simulink model "simulink_motor"  (R2018b)
settings: Solver=VariableStepAuto  StartTime=0.0  StopTime=100  RelTol=1e-6
settings Model: Creator=aland  LastModifiedBy=aland

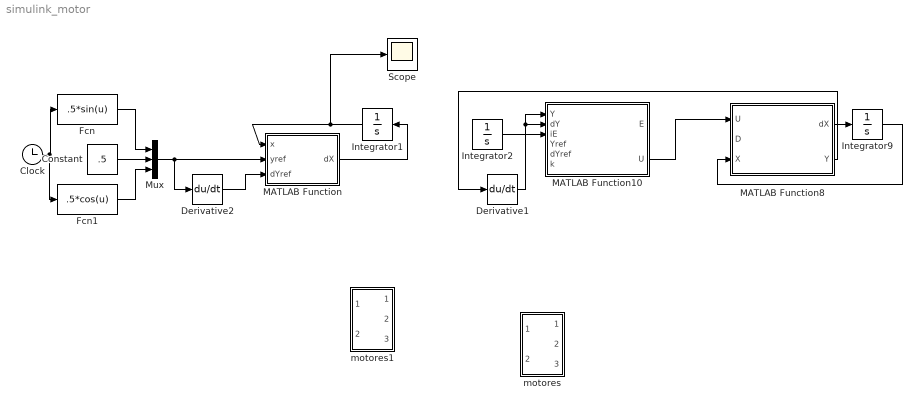
== system simulink_motor ==
  Clock : Clock
      settings: Decimation=1000
  Constant : Constant  Value=.5
  Derivative1 : Derivative
  Derivative2 : Derivative
  Fcn : Fcn  Expr=.5*sin(u)
  Fcn1 : Fcn  Expr=.5*cos(u)
  Integrator1 : Integrator  InitialCondition=[0 0 0 0 0 0 0 .148 0 1.2385]  UpperSaturationLimit=4  LowerSaturationLimit=-4
  Integrator2 : Integrator  InitialCondition=[0 0]
  Integrator9 : Integrator  InitialCondition=[0 0]
  MATLAB Function : MATLAB Function  TreatAsAtomicUnit=on
  MATLAB Function10 : MATLAB Function  TreatAsAtomicUnit=on
  MATLAB Function8 : MATLAB Function  TreatAsAtomicUnit=on
  Mux : Mux  Inputs=3
  Scope : Scope
  motores : Subsystem  InitFcn=robot_init
  motores1 : Subsystem  InitFcn=robot_init
  wires:
  Fcn/1 -> Mux/1
  Constant/1 -> Mux/2
  Fcn1/1 -> Mux/3
  Mux/1 -> Derivative2/1, MATLAB Function/2(yref)
  Derivative2/1 -> MATLAB Function/3(dYref)
  MATLAB Function/1(dX) -> Integrator1/1
  Integrator1/1 -> Scope/1, MATLAB Function/1(x)
  Clock/1 -> Fcn1/1, Fcn/1
  MATLAB Function8/1(dX) -> Integrator9/1
  MATLAB Function10/2(U) -> MATLAB Function8/1(U)
  Integrator9/1 -> MATLAB Function8/3(X)
  MATLAB Function8/2(Y) -> Derivative1/1
  Derivative1/1 -> MATLAB Function10/1(Y), MATLAB Function10/2(dY)
  Integrator2/1 -> MATLAB Function10/3(iE)

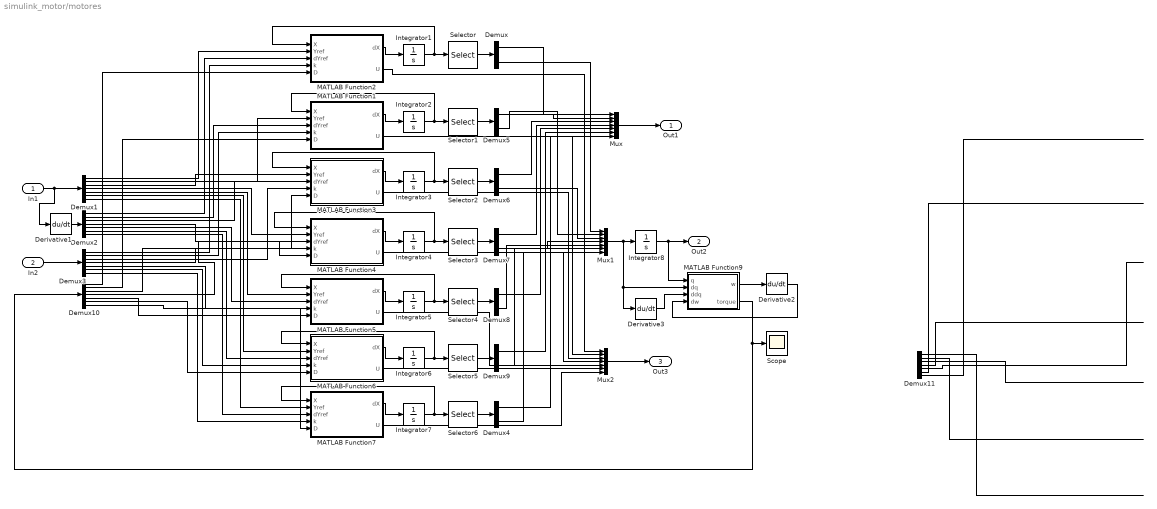
== system simulink_motor/motores ==
  In1 : Inport
  In2 : Inport  Port=2
  Demux{,4..9} (7 alike) : Demux  Outputs=2
  Demux{1..2,10..11} (4 alike) : Demux  Outputs=7
  Demux3 : Demux  Outputs=[3 3 3 3 3 3 3]
  Derivative1 : Derivative
  Derivative2 : Derivative
  Derivative3 : Derivative
  Integrator{1..7} (7 alike) : Integrator  InitialCondition=[0 0 0]
  Integrator8 : Integrator  InitialCondition=[0 0 0 0 0 0 0]  UpperSaturationLimit=4  LowerSaturationLimit=-4
  MATLAB Function1 : MATLAB Function  TreatAsAtomicUnit=on
  MATLAB Function2 : MATLAB Function  TreatAsAtomicUnit=on
  MATLAB Function3 : MATLAB Function  TreatAsAtomicUnit=on
  MATLAB Function4 : MATLAB Function  TreatAsAtomicUnit=on
  MATLAB Function5 : MATLAB Function  TreatAsAtomicUnit=on
  MATLAB Function6 : MATLAB Function  TreatAsAtomicUnit=on
  MATLAB Function7 : MATLAB Function  TreatAsAtomicUnit=on
  MATLAB Function9 : MATLAB Function  TreatAsAtomicUnit=on
      mask init:
      | m = 0;
  Mux : Mux  Inputs=7
  Mux1 : Mux  Inputs=7
  Mux2 : Mux  Inputs=7
  Scope : Scope
  Selector{,1..6} (7 alike) : Selector  InputPortWidth=3  IndexOptions=Index vector (dialog)  Indices=[2:3]  OutputSizes=1
  Out1 : Outport
  Out2 : Outport  Port=2
  Out3 : Outport  Port=3
  wires:
  In2/1 -> Demux3/1
  Demux4/2 -> Mux1/7
  Demux3/6 -> MATLAB Function6/4(k)
  Demux3/2 -> MATLAB Function1/4(k)
  Demux3/4 -> MATLAB Function4/4(k)
  Integrator4/1 -> Selector3/1, MATLAB Function4/1(X)
  Demux5/2 -> Mux1/2
  MATLAB Function3/1(dX) -> Integrator3/1
  MATLAB Function6/1(dX) -> Integrator6/1
  Demux5/1 -> Mux/2
  Integrator2/1 -> Selector1/1, MATLAB Function1/1(X)
  Integrator1/1 -> MATLAB Function2/1(X), Selector/1
  Demux2/7 -> MATLAB Function7/3(dYref)
  MATLAB Function4/1(dX) -> Integrator4/1
  Demux2/1 -> MATLAB Function2/3(dYref)
  Demux3/5 -> MATLAB Function5/4(k)
  Demux1/5 -> MATLAB Function5/2(Yref)
  Integrator6/1 -> Selector5/1, MATLAB Function6/1(X)
  Demux2/3 -> MATLAB Function3/3(dYref)
  Integrator3/1 -> Selector2/1, MATLAB Function3/1(X)
  Demux2/5 -> MATLAB Function5/3(dYref)
  Demux1/4 -> MATLAB Function4/2(Yref)
  MATLAB Function1/1(dX) -> Integrator2/1
  Demux1/6 -> MATLAB Function6/2(Yref)
  Demux7/1 -> Mux/4
  MATLAB Function5/1(dX) -> Integrator5/1
  Integrator5/1 -> Selector4/1, MATLAB Function5/1(X)
  Demux6/1 -> Mux/3
  MATLAB Function7/1(dX) -> Integrator7/1
  Demux1/7 -> MATLAB Function7/2(Yref)
  Demux3/7 -> MATLAB Function7/4(k)
  Demux9/2 -> Mux1/6
  Integrator7/1 -> Selector6/1, MATLAB Function7/1(X)
  Demux1/1 -> MATLAB Function2/2(Yref)
  Demux8/2 -> Mux1/5
  Demux6/2 -> Mux1/3
  Demux3/3 -> MATLAB Function3/4(k)
  Demux7/2 -> Mux1/4
  Demux2/6 -> MATLAB Function6/3(dYref)
  Demux/2 -> Mux1/1
  Demux9/1 -> Mux/6
  Demux8/1 -> Mux/5
  Demux1/2 -> MATLAB Function1/2(Yref)
  Demux/1 -> Mux/1
  Demux1/3 -> MATLAB Function3/2(Yref)
  MATLAB Function2/1(dX) -> Integrator1/1
  Demux3/1 -> MATLAB Function2/4(k)
  Demux2/4 -> MATLAB Function4/3(dYref)
  Demux4/1 -> Mux/7
  Demux2/2 -> MATLAB Function1/3(dYref)
  Mux/1 -> Out1/1
  In1/1 -> Derivative1/1, Demux1/1
  Selector/1 -> Demux/1
  Selector1/1 -> Demux5/1
  Selector2/1 -> Demux6/1
  Selector3/1 -> Demux7/1
  Selector4/1 -> Demux8/1
  Selector5/1 -> Demux9/1
  Selector6/1 -> Demux4/1
  Derivative1/1 -> Demux2/1
  Mux2/1 -> Out3/1
  MATLAB Function2/2(U) -> Mux2/1
  MATLAB Function1/2(U) -> Mux2/2
  MATLAB Function4/2(U) -> Mux2/4
  MATLAB Function3/2(U) -> Mux2/3
  MATLAB Function6/2(U) -> Mux2/6
  MATLAB Function5/2(U) -> Mux2/5
  MATLAB Function7/2(U) -> Mux2/7
  Mux1/1 -> MATLAB Function9/2(dq), Derivative3/1, Integrator8/1
  Integrator8/1 -> MATLAB Function9/1(q), Out2/1
  MATLAB Function9/1(w) -> Derivative2/1
  Derivative2/1 -> MATLAB Function9/4(dw)
  Derivative3/1 -> MATLAB Function9/3(ddq)
  Demux11/1 -> ?
  Demux11/2 -> ?
  Demux11/3 -> ?
  Demux11/4 -> ?
  Demux11/5 -> ?
  Demux11/7 -> ?
  Demux11/6 -> ?
  Demux10/4 -> MATLAB Function4/5(D)
  Demux10/7 -> MATLAB Function7/5(D)
  Demux10/1 -> MATLAB Function2/5(D)
  Demux10/5 -> MATLAB Function5/5(D)
  Demux10/2 -> MATLAB Function1/5(D)
  Demux10/6 -> MATLAB Function6/5(D)
  MATLAB Function9/2(torque) -> Scope/1, Demux10/1
  Demux10/3 -> MATLAB Function3/5(D)

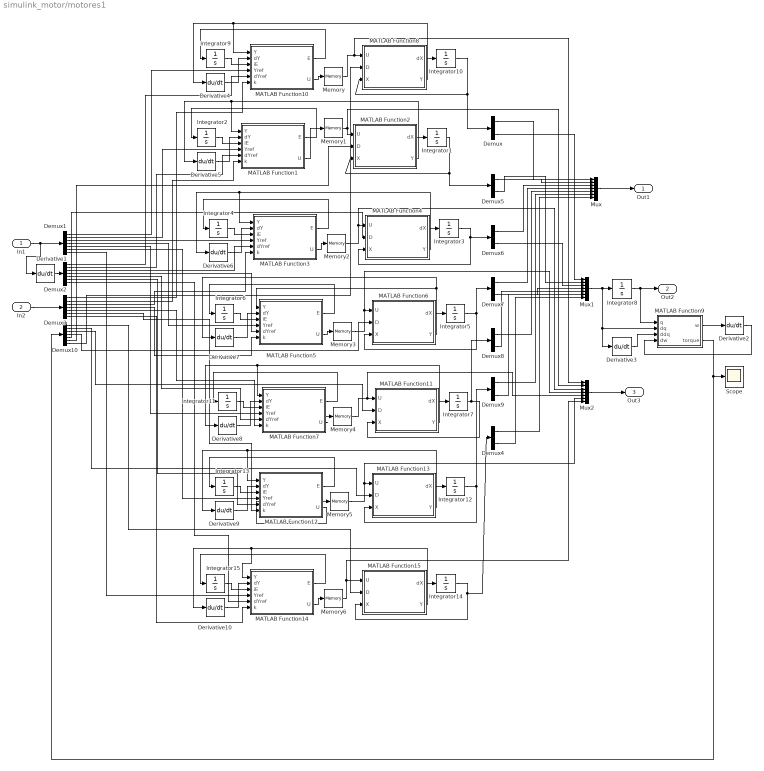
== system simulink_motor/motores1 ==
  In1 : Inport
  In2 : Inport  Port=2
  Demux{,4..9} (7 alike) : Demux  Outputs=2
  Demux1 : Demux  Outputs=7
  Demux10 : Demux  Outputs=7
  Demux2 : Demux  Outputs=7
  Demux3 : Demux  Outputs=[3 3 3 3 3 3 3]
  Derivative{1..10} (10 alike) : Derivative
  Integrator{1,3,5,7,10,12,14} (7 alike) : Integrator  InitialCondition=[0 0]
  Integrator{2,4,6,9,11,13,15} (7 alike) : Integrator
  Integrator8 : Integrator  InitialCondition=[0 0 0 0 0 0 0]  UpperSaturationLimit=4  LowerSaturationLimit=-4
  MATLAB Function1 : MATLAB Function  TreatAsAtomicUnit=on
  MATLAB Function10 : MATLAB Function  TreatAsAtomicUnit=on
  MATLAB Function11 : MATLAB Function  TreatAsAtomicUnit=on
  MATLAB Function12 : MATLAB Function  TreatAsAtomicUnit=on
  MATLAB Function13 : MATLAB Function  TreatAsAtomicUnit=on
  MATLAB Function14 : MATLAB Function  TreatAsAtomicUnit=on
  MATLAB Function15 : MATLAB Function  TreatAsAtomicUnit=on
  MATLAB Function2 : MATLAB Function  TreatAsAtomicUnit=on
  MATLAB Function3 : MATLAB Function  TreatAsAtomicUnit=on
  MATLAB Function4 : MATLAB Function  TreatAsAtomicUnit=on
  MATLAB Function5 : MATLAB Function  TreatAsAtomicUnit=on
  MATLAB Function6 : MATLAB Function  TreatAsAtomicUnit=on
  MATLAB Function7 : MATLAB Function  TreatAsAtomicUnit=on
  MATLAB Function8 : MATLAB Function  TreatAsAtomicUnit=on
  MATLAB Function9 : MATLAB Function  TreatAsAtomicUnit=on
      mask init:
      | m = 0;
  Memory{,1..6} (7 alike) : Memory
  Mux : Mux  Inputs=7
  Mux1 : Mux  Inputs=7
  Mux2 : Mux  Inputs=7
  Scope : Scope
  Out1 : Outport
  Out2 : Outport  Port=2
  Out3 : Outport  Port=3
  wires:
  In2/1 -> Demux3/1
  Demux4/2 -> Mux1/7
  Demux5/2 -> Mux1/2
  Demux5/1 -> Mux/2
  Demux7/1 -> Mux/4
  Demux6/1 -> Mux/3
  Demux9/2 -> Mux1/6
  Demux8/2 -> Mux1/5
  Demux6/2 -> Mux1/3
  Demux7/2 -> Mux1/4
  Demux/2 -> Mux1/1
  Demux9/1 -> Mux/6
  Demux8/1 -> Mux/5
  Demux/1 -> Mux/1
  Demux4/1 -> Mux/7
  Mux/1 -> Out1/1
  In1/1 -> Derivative1/1, Demux1/1
  Integrator1/1 -> Demux5/1, MATLAB Function2/3(X)
  Integrator3/1 -> Demux6/1, MATLAB Function4/3(X)
  Integrator5/1 -> Demux7/1, MATLAB Function6/3(X)
  Integrator12/1 -> Demux9/1, MATLAB Function13/3(X)
  Integrator7/1 -> Demux8/1, MATLAB Function11/3(X)
  Derivative1/1 -> Demux2/1
  Mux2/1 -> Out3/1
  Mux1/1 -> MATLAB Function9/2(dq), Derivative3/1, Integrator8/1
  Integrator8/1 -> MATLAB Function9/1(q), Out2/1
  MATLAB Function9/1(w) -> Derivative2/1
  Derivative2/1 -> MATLAB Function9/4(dw)
  Derivative3/1 -> MATLAB Function9/3(ddq)
  MATLAB Function9/2(torque) -> Scope/1, Demux10/1
  MATLAB Function8/1(dX) -> Integrator10/1
  MATLAB Function8/2(Y) -> MATLAB Function10/1(Y), Derivative4/1
  Derivative4/1 -> MATLAB Function10/2(dY)
  Integrator9/1 -> MATLAB Function10/3(iE)
  Integrator10/1 -> Demux/1, MATLAB Function8/3(X)
  MATLAB Function10/1(E) -> Integrator9/1
  Derivative5/1 -> MATLAB Function1/2(dY)
  Integrator2/1 -> MATLAB Function1/3(iE)
  MATLAB Function2/2(Y) -> MATLAB Function1/1(Y), Derivative5/1
  MATLAB Function2/1(dX) -> Integrator1/1
  MATLAB Function1/1(E) -> Integrator2/1
  Derivative6/1 -> MATLAB Function3/2(dY)
  Integrator4/1 -> MATLAB Function3/3(iE)
  MATLAB Function4/2(Y) -> MATLAB Function3/1(Y), Derivative6/1
  MATLAB Function4/1(dX) -> Integrator3/1
  MATLAB Function3/1(E) -> Integrator4/1
  Derivative7/1 -> MATLAB Function5/2(dY)
  Integrator6/1 -> MATLAB Function5/3(iE)
  MATLAB Function6/2(Y) -> MATLAB Function5/1(Y), Derivative7/1
  MATLAB Function6/1(dX) -> Integrator5/1
  MATLAB Function5/1(E) -> Integrator6/1
  Derivative8/1 -> MATLAB Function7/2(dY)
  Integrator11/1 -> MATLAB Function7/3(iE)
  MATLAB Function11/2(Y) -> MATLAB Function7/1(Y), Derivative8/1
  MATLAB Function11/1(dX) -> Integrator7/1
  MATLAB Function7/1(E) -> Integrator11/1
  Derivative9/1 -> MATLAB Function12/2(dY)
  Integrator13/1 -> MATLAB Function12/3(iE)
  MATLAB Function13/2(Y) -> MATLAB Function12/1(Y), Derivative9/1
  MATLAB Function13/1(dX) -> Integrator12/1
  MATLAB Function12/1(E) -> Integrator13/1
  Derivative10/1 -> MATLAB Function14/2(dY)
  Integrator15/1 -> MATLAB Function14/3(iE)
  MATLAB Function15/2(Y) -> MATLAB Function14/1(Y), Derivative10/1
  Integrator14/1 -> Demux4/1, MATLAB Function15/3(X)
  MATLAB Function15/1(dX) -> Integrator14/1
  MATLAB Function14/1(E) -> Integrator15/1
  Demux1/2 -> MATLAB Function1/4(Yref)
  Demux1/1 -> MATLAB Function10/4(Yref)
  Demux1/3 -> MATLAB Function3/4(Yref)
  Demux1/4 -> MATLAB Function5/4(Yref)
  Demux2/1 -> MATLAB Function10/5(dYref)
  Demux2/2 -> MATLAB Function1/5(dYref)
  Demux2/3 -> MATLAB Function3/5(dYref)
  Demux2/4 -> MATLAB Function5/5(dYref)
  Demux3/1 -> MATLAB Function10/6(k)
  Demux3/2 -> MATLAB Function1/6(k)
  Demux3/4 -> MATLAB Function5/6(k)
  Demux3/3 -> MATLAB Function3/6(k)
  Demux1/5 -> MATLAB Function7/4(Yref)
  Demux2/5 -> MATLAB Function7/5(dYref)
  Demux1/6 -> MATLAB Function12/4(Yref)
  Demux1/7 -> MATLAB Function14/4(Yref)
  Demux2/6 -> MATLAB Function12/5(dYref)
  Demux2/7 -> MATLAB Function14/5(dYref)
  Demux3/5 -> MATLAB Function7/6(k)
  Demux3/6 -> MATLAB Function12/6(k)
  Demux3/7 -> MATLAB Function14/6(k)
  MATLAB Function10/2(U) -> Memory/1
  Memory/1 -> Mux2/1, MATLAB Function8/1(U)
  MATLAB Function1/2(U) -> Memory1/1
  Memory1/1 -> MATLAB Function2/1(U), Mux2/2
  MATLAB Function3/2(U) -> Memory2/1
  MATLAB Function5/2(U) -> Memory3/1
  Memory3/1 -> Mux2/4, MATLAB Function6/1(U)
  MATLAB Function7/2(U) -> Memory4/1
  Memory4/1 -> Mux2/5, MATLAB Function11/1(U)
  MATLAB Function12/2(U) -> Memory5/1
  Memory5/1 -> Mux2/6, MATLAB Function13/1(U)
  Memory2/1 -> Mux2/3, MATLAB Function4/1(U)
  Memory6/1 -> Mux2/7, MATLAB Function15/1(U)
  MATLAB Function14/2(U) -> Memory6/1
  Demux10/7 -> MATLAB Function8/2(D)
  Demux10/6 -> MATLAB Function2/2(D)
  Demux10/5 -> MATLAB Function4/2(D)
  Demux10/4 -> MATLAB Function6/2(D)
  Demux10/3 -> MATLAB Function11/2(D)
  Demux10/1 -> MATLAB Function15/2(D)
  Demux10/2 -> MATLAB Function13/2(D)

== matlab function simulink_motor/motores/MATLAB Function2 ==
  data: X input; dX output; Yref input; dYref input; k input; U output; D input
function [dX,U]= motor_pid(X, Yref, dYref, k, D)

%MATRICES DEL MOTOR
Ra = 11.24;
La = 2.713e-3;
Kb = 14.87e-3;
Kt = Kb;
bm = 2.01e-6;
Jm = 2779.56e-9;

A = [-Ra/La -Kb/La;Kt/Jm -bm/Jm];
B = [1/La;0];
C = [0 1];

%CONTROLADOR PID
E = Yref - C*X(2:3);
dE = dYref - C*A*X(2:3);

U = k(1)*E + k(2)*X(1) + k(3)*dE;

if(U > 48)
    U = 48;
    
elseif(U < -48)
    U = -48;
end

dX = [E; A*X(2:3) + B*U];

== matlab function simulink_motor/MATLAB Function ==
  data: x input; dX output; yref input; dYref input
function dX = simulink_jacobiano(x, yref,dYref)

Ke = -5;

%Parametros del sistema
d = [0.2703 0 0.3644 0 0.3743 0 0.2295]; %metros
a = [0.069 0 0.069 0 0.01 0 0]; %metros
alpha = [-pi/2 pi/2 -pi/2 pi/2 -pi/2 pi/2 0]; %radianes

T = D_H(x(1:7),a,alpha,d,0,7);
J = jacobiano(T);
Jv = J(4:6,:);

e = yref - T{1,7}(1:3,4);
U = pinv(Jv)*(dYref - Ke*e);
    
%ODE's
dX = [U;Jv*U];

== matlab function simulink_motor/motores/MATLAB Function1 ==
  data: X input; dX output; Yref input; dYref input; k input; U output; D input
function [dX,U]= motor_pid(X, Yref, dYref, k, D)

%MATRICES DEL MOTOR
Ra = 11.24;
La = 2.713e-3;
Kb = 14.87e-3;
Kt = Kb;
bm = 2.01e-6;
Jm = 2779.56e-9;

A = [-Ra/La -Kb/La;Kt/Jm -bm/Jm];
B = [1/La;0];
C = [0 1];

%CONTROLADOR PID
E = Yref - C*X(2:3);
dE = dYref - C*A*X(2:3);

U = k(1)*E + k(2)*X(1) + k(3)*dE;

if(U > 48)
    U = 48;
    
elseif(U < -48)
    U = -48;
end

dX = [E; A*X(2:3) + B*U];

== matlab function simulink_motor/motores/MATLAB Function3 ==
  data: X input; dX output; Yref input; dYref input; k input; U output; D input
function [dX,U]= motor_pid(X, Yref, dYref, k, D)

%MATRICES DEL MOTOR
Ra = 11.24;
La = 2.713e-3;
Kb = 14.87e-3;
Kt = Kb;
bm = 2.01e-6;
Jm = 2779.56e-9;

A = [-Ra/La -Kb/La;Kt/Jm -bm/Jm];
B = [1/La;0];
C = [0 1];

%CONTROLADOR PID
E = Yref - C*X(2:3);
dE = dYref - C*A*X(2:3);

U = k(1)*E + k(2)*X(1) + k(3)*dE;

if(U > 48)
    U = 48;
    
elseif(U < -48)
    U = -48;
end

dX = [E; A*X(2:3) + B*U];

== matlab function simulink_motor/motores/MATLAB Function4 ==
  data: X input; dX output; Yref input; dYref input; k input; U output; D input
function [dX,U]= motor_pid(X, Yref, dYref, k, D)

%MATRICES DEL MOTOR
Ra = 11.24;
La = 2.713e-3;
Kb = 14.87e-3;
Kt = Kb;
bm = 2.01e-6;
Jm = 2779.56e-9;

A = [-Ra/La -Kb/La;Kt/Jm -bm/Jm];
B = [1/La;0];
C = [0 1];

%CONTROLADOR PID
E = Yref - C*X(2:3);
dE = dYref - C*A*X(2:3);

U = k(1)*E + k(2)*X(1) + k(3)*dE;

if(U > 48)
    U = 48;
    
elseif(U < -48)
    U = -48;
end

dX = [E; A*X(2:3) + B*U];

== matlab function simulink_motor/motores/MATLAB Function5 ==
  data: X input; dX output; Yref input; dYref input; k input; U output; D input
function [dX,U]= motor_pid(X, Yref, dYref, k, D)

%MATRICES DEL MOTOR
Ra = 11.24;
La = 2.713e-3;
Kb = 14.87e-3;
Kt = Kb;
bm = 2.01e-6;
Jm = 2779.56e-9;

A = [-Ra/La -Kb/La;Kt/Jm -bm/Jm];
B = [1/La;0];
C = [0 1];

%CONTROLADOR PID
E = Yref - C*X(2:3);
dE = dYref - C*A*X(2:3);

U = k(1)*E + k(2)*X(1) + k(3)*dE;

if(U > 48)
    U = 48;
    
elseif(U < -48)
    U = -48;
end

dX = [E; A*X(2:3) + B*U];

== matlab function simulink_motor/motores/MATLAB Function6 ==
  data: X input; dX output; Yref input; dYref input; k input; U output; D input
function [dX,U]= motor_pid(X, Yref, dYref, k, D)

%MATRICES DEL MOTOR
Ra = 11.24;
La = 2.713e-3;
Kb = 14.87e-3;
Kt = Kb;
bm = 2.01e-6;
Jm = 2779.56e-9;

A = [-Ra/La -Kb/La;Kt/Jm -bm/Jm];
B = [1/La;0];
C = [0 1];

%CONTROLADOR PID
E = Yref - C*X(2:3);
dE = dYref - C*A*X(2:3);

U = k(1)*E + k(2)*X(1) + k(3)*dE;

if(U > 48)
    U = 48;
    
elseif(U < -48)
    U = -48;
end

dX = [E; A*X(2:3) + B*U];

== matlab function simulink_motor/motores/MATLAB Function7 ==
  data: X input; dX output; Yref input; dYref input; k input; U output; D input
function [dX,U]= motor_pid(X, Yref, dYref, k, D)

%MATRICES DEL MOTOR
Ra = 11.24;
La = 2.713e-3;
Kb = 14.87e-3;
Kt = Kb;
bm = 2.01e-6;
Jm = 2779.56e-9;

A = [-Ra/La -Kb/La;Kt/Jm -bm/Jm];
B = [1/La;0];
C = [0 1];

%CONTROLADOR PID
E = Yref - C*X(2:3);
dE = dYref - C*A*X(2:3);

U = k(1)*E + k(2)*X(1) + k(3)*dE;

if(U > 48)
    U = 48;
    
elseif(U < -48)
    U = -48;
end

dX = [E; A*X(2:3) + B*U];

== matlab function simulink_motor/motores1/MATLAB Function1 ==
  data: E output; Y input; dY input; iE input; U output; Yref input; dYref input; k input
function [E,U] = PID(Y,dY,iE,Yref,dYref,k)

E = Yref - Y;
dE = dYref - dY;

U = k(1)*E + k(2)*iE + k(3)*dE;

== matlab function simulink_motor/motores/MATLAB Function9 ==
  data: w output; q input; dq input; torque output; ddq input; dw input
function [w,torque] = fcn(q, dq, ddq, dw)

d = [0.2703 0 0.3644 0 0.3743 0 0.2295]; %metros
a = [0.069 0 0.069 0 0.01 0 0]; %matros
alpha = [-pi/2 pi/2 -pi/2 pi/2 -pi/2 pi/2 0]; %radianes
m = [5.70044 3.22698 4.31272 2.07206 2.24665 1.60879 0.54218]; %kg

xc = [-0.05117 0.00269 -0.07176 0.00159 -0.01168 0.00697 0.005137]; %metros
yc = [0.07908 -0.00529 0.08149 -0.01117 0.13111 0.006 0.0009572];
zc = [0.00086 0.06845 0.00132 0.02618 0.0046 0.06048 0.0-6682];

%Tensores de inercia (kg*m^2)
Ixx = [0.047091023 0.027885975 0.026617336 0.013182279 0.016677428 0.007005379 0.000816214];
Iyy = [0.035959884 0.020787492 0.012480083 0.00926852 0.003746311 0.005527552 0.000873501];
Izz = [0.037669765 0.011752094 0.028443552 0.007115827 0.016754573 0.003876072 0.000549415];
Ixy = [-0.0061487 -0.00018822 -0.003921899 -0.000196634 -0.000186576 0.000153481 0.00012844];
Iyx = [-0.0061487 -0.00018822 -0.003921899 -0.000196634 -0.000186576 0.000153481 0.00012844];
Iyz = [-0.000780869 0.002076758 -0.001083893 0.000745949 0.000647324 -0.00021115 0.000105773];
Izy = [-0.000780869 0.002076758 -0.001083893 0.000745949 0.000647324 -0.00021115 0.000105773];
Ixz = [0.000127876 -0.000300964 0.000292706 0.000360362 0.000184037 -0.000443848 0.000189699];
Izx = [0.000127876 -0.000300964 0.000292706 0.000360362 0.000184037 -0.000443848 0.000189699];

Ti = D_H(q,a,alpha,d,0,7);
rici = zeros(3,7);
rmci = zeros(3,7);
rimi = zeros(3,7);

for i = 1:7
    rici(:,i) = Ti{i}(1:3,4)- [xc(i);yc(i);zc(i)];
end

for i = 1:6
    rmci(:,i) = Ti{i + 1}(1:3,4)- Ti{i}(1:3,4) - [xc(i);yc(i);zc(i)];
end

for i = 1:6
    rimi(:,i) = Ti{i + 1}(1:3,4) - Ti{i}(1:3,4);
end

T0 = D_H(q,a,alpha,d,0,7);

w = zeros(3,7);
aw = zeros(3,7);
ac = zeros(3,7);
ae = zeros(3,7);
f = zeros(3,7);
g = zeros(3,7);
Tq = zeros(3,7);
torque = zeros(7,1);

%w1
Ri = Ti{1}(1:3,1:3);
Z0 = [0;0;1];
bi = Ri'*Z0;
w(:,1) = bi*dq(1);
aw(:,1) = bi*ddq(1) + cross(w(:,1),bi*dq(1));
ae(:,1) = cross(dw(:,1),rimi(:,1)) + cross(w(:,1),cross(w(:,1),rimi(:,1)));
ac(:,1) = cross(dw(:,1),rici(:,1)) + cross(w(:,1),cross(w(:,1),rici(:,1)));
g(:,1) = -Ri'*9.78*[0;0;1];

for i = 2:7
   Ri = Ti{i}(1:3,1:3); 
   Rmi = [dot(Ti{i}(1,4),Ti{i-1}(1,4)) dot(Ti{i}(2,4),Ti{i-1}(1,4)) dot(Ti{i}(3,4),Ti{i-1}(1,4));...
       dot(Ti{i}(1,4),Ti{i-1}(2,4)) dot(Ti{i}(2,4),Ti{i-1}(2,4)) dot(Ti{i}(3,4),Ti{i-1}(2,4));...
       dot(Ti{i}(1,4),Ti{i-1}(3,4)) dot(Ti{i}(2,4),Ti{i-1}(3,4)) dot(Ti{i}(3,4),Ti{i-1}(3,4))]';
   bi = Ri'*Ti{i - 1}(1:3,3);
   w(:,i) = Rmi'*w(:,i-1) + bi*dq(i);
   aw(:,i) = Rmi'*aw(:,i-1) +bi*ddq(i) + cross(w(:,i),bi*dq(i));
   ae(:,i) = Rmi'*ae(:,i-1) + cross(dw(:,i),rimi(:,i)) + cross(w(:,i),cross(w(:,i),rimi(:,i)));
   ac(:,i) = Rmi'*ac(:,i-1) + cross(dw(:,i),rici(:,i)) + cross(w(:,i),cross(w(:,i),rici(:,i)));
   g(:,i) = -Ri'*9.78*[0;0;1];
end

%f7
f(:,7) = m(7)*ac(:,7) - m(7)*g(:,7);
I = [Ixx(7) Ixy(7) Ixz(7);Iyx(7) Iyy(7) Iyz(7);Izx(7) Izy(7) Izz(7)];
Tq(:,7) = - cross(f(:,7),rici(:,7)) + aw(:,7) + cross(w(:,7),I*w(:,7));
torque(7) = sqrt(Tq(1,7)^2 + Tq(2,7)^2 + Tq(3,7)^2);

for i = 6:-1:1
    Rmi = [dot(Ti{i + 1}(1,4),Ti{i}(1,4)) dot(Ti{i + 1}(2,4),Ti{i}(1,4)) dot(Ti{i+1}(3,4),Ti{i}(1,4));...
       dot(Ti{i+1}(1,4),Ti{i}(2,4)) dot(Ti{i+1}(2,4),Ti{i}(2,4)) dot(Ti{i+1}(3,4),Ti{i}(2,4));...
       dot(Ti{i+1}(1,4),Ti{i}(3,4)) dot(Ti{i+1}(2,4),Ti{i}(3,4)) dot(Ti{i+1}(3,4),Ti{i}(3,4))]';
   I = [Ixx(i) Ixy(i) Ixz(i);Iyx(i) Iyy(i) Iyz(i);Izx(i) Izy(i) Izz(i)];
   f(:,i) = Rmi*f(:,i+1) + m(i)*ac(:,i) - m(i)*g(:,i);
   Tq(:,i) = Rmi*Tq(:,i+1) - cross(f(:,i),rici(:,i)) + cross(Rmi*f(:,i+1),rmci(:,i)) + aw(:,i) + cross(w(:,i),I*w(:,i));
   torque(i) = sqrt(Tq(1,i)^2 + Tq(2,i)^2 + Tq(3,i)^2);
end

== matlab function simulink_motor/motores1/MATLAB Function10 ==
  data: E output; Y input; dY input; iE input; U output; Yref input; dYref input; k input
function [E,U] = PID(Y,dY,iE,Yref,dYref,k)

E = Yref - Y;
dE = dYref - dY;

U = k(1)*E + k(2)*iE + k(3)*dE;

== matlab function simulink_motor/motores1/MATLAB Function11 ==
  data: U input; D input; dX output; Y output; X input
function [dX,Y]= motor_modelo(U,D,X)

%MATRICES DEL MOTOR
Ra = 11.24;
La = 2.713e-3;
Kb = 14.87e-3;
Kt = Kb;
bm = 2.01e-6;
Jm = 2779.56e-9;

A = [-Ra/La -Kb/La;Kt/Jm -bm/Jm];
B = [1/La;0];
C = [0 1];

%CONTROLADOR PID
dX = [A*X + B*U];
Y = [C*X + D*U];

== matlab function simulink_motor/motores1/MATLAB Function12 ==
  data: E output; Y input; dY input; iE input; U output; Yref input; dYref input; k input
function [E,U] = PID(Y,dY,iE,Yref,dYref,k)

E = Yref - Y;
dE = dYref - dY;

U = k(1)*E + k(2)*iE + k(3)*dE;

== matlab function simulink_motor/motores1/MATLAB Function13 ==
  data: U input; D input; dX output; Y output; X input
function [dX,Y]= motor_modelo(U,D,X)

%MATRICES DEL MOTOR
Ra = 11.24;
La = 2.713e-3;
Kb = 14.87e-3;
Kt = Kb;
bm = 2.01e-6;
Jm = 2779.56e-9;

A = [-Ra/La -Kb/La;Kt/Jm -bm/Jm];
B = [1/La;0];
C = [0 1];

%CONTROLADOR PID
dX = [A*X + B*U];
Y = [C*X + D*U];

== matlab function simulink_motor/motores1/MATLAB Function14 ==
  data: E output; Y input; dY input; iE input; U output; Yref input; dYref input; k input
function [E,U] = PID(Y,dY,iE,Yref,dYref,k)

E = Yref - Y;
dE = dYref - dY;

U = k(1)*E + k(2)*iE + k(3)*dE;

== matlab function simulink_motor/motores1/MATLAB Function15 ==
  data: U input; D input; dX output; Y output; X input
function [dX,Y]= motor_modelo(U,D,X)

%MATRICES DEL MOTOR
Ra = 11.24;
La = 2.713e-3;
Kb = 14.87e-3;
Kt = Kb;
bm = 2.01e-6;
Jm = 2779.56e-9;

A = [-Ra/La -Kb/La;Kt/Jm -bm/Jm];
B = [1/La;0];
C = [0 1];

%CONTROLADOR PID
dX = [A*X + B*U];
Y = [C*X + D*U];

== matlab function simulink_motor/motores1/MATLAB Function2 ==
  data: U input; D input; dX output; Y output; X input
function [dX,Y]= motor_modelo(U,D,X)

%MATRICES DEL MOTOR
Ra = 11.24;
La = 2.713e-3;
Kb = 14.87e-3;
Kt = Kb;
bm = 2.01e-6;
Jm = 2779.56e-9;

A = [-Ra/La -Kb/La;Kt/Jm -bm/Jm];
B = [1/La;0];
C = [0 1];

%CONTROLADOR PID
dX = [A*X + B*U];
Y = [C*X + D*U];

== matlab function simulink_motor/MATLAB Function8 ==
  data: U input; D input; dX output; Y output; X input
function [dX,Y]= motor_modelo(U,D,X)

%MATRICES DEL MOTOR
Ra = 11.24;
La = 2.713e-3;
Kb = 14.87e-3;
Kt = Kb;
bm = 2.01e-6;
Jm = 2779.56e-9;

A = [-Ra/La -Kb/La;Kt/Jm -bm/Jm];
B = [1/La;0];
C = [0 1];

%CONTROLADOR PID
dX = [A*X(2:3) + B*U];
Y = [C*X + D*U];

== matlab function simulink_motor/MATLAB Function10 ==
  data: E output; Y input; dY input; iE input; U output; Yref input; dYref input; k input
function [E,U] = PID(Y,dY,iE,Yref,dYref,k)

E = Yref - Y;
dE = dYref - dY;

U = k(1)*E + k(2)*iE + k(3)*dE;

if(U > 48)
    U = 48;
    
elseif(U < -48)
    U = -48;
end

== matlab function simulink_motor/motores1/MATLAB Function3 ==
  data: E output; Y input; dY input; iE input; U output; Yref input; dYref input; k input
function [E,U] = PID(Y,dY,iE,Yref,dYref,k)

E = Yref - Y;
dE = dYref - dY;

U = k(1)*E + k(2)*iE + k(3)*dE;

== matlab function simulink_motor/motores1/MATLAB Function4 ==
  data: U input; D input; dX output; Y output; X input
function [dX,Y]= motor_modelo(U,D,X)

%MATRICES DEL MOTOR
Ra = 11.24;
La = 2.713e-3;
Kb = 14.87e-3;
Kt = Kb;
bm = 2.01e-6;
Jm = 2779.56e-9;

A = [-Ra/La -Kb/La;Kt/Jm -bm/Jm];
B = [1/La;0];
C = [0 1];

%CONTROLADOR PID
dX = [A*X + B*U];
Y = [C*X + D*U];

== matlab function simulink_motor/motores1/MATLAB Function5 ==
  data: E output; Y input; dY input; iE input; U output; Yref input; dYref input; k input
function [E,U] = PID(Y,dY,iE,Yref,dYref,k)

E = Yref - Y;
dE = dYref - dY;

U = k(1)*E + k(2)*iE + k(3)*dE;

== matlab function simulink_motor/motores1/MATLAB Function6 ==
  data: U input; D input; dX output; Y output; X input
function [dX,Y]= motor_modelo(U,D,X)

%MATRICES DEL MOTOR
Ra = 11.24;
La = 2.713e-3;
Kb = 14.87e-3;
Kt = Kb;
bm = 2.01e-6;
Jm = 2779.56e-9;

A = [-Ra/La -Kb/La;Kt/Jm -bm/Jm];
B = [1/La;0];
C = [0 1];

%CONTROLADOR PID
dX = [A*X + B*U];
Y = [C*X + D*U];

== matlab function simulink_motor/motores1/MATLAB Function7 ==
  data: E output; Y input; dY input; iE input; U output; Yref input; dYref input; k input
function [E,U] = PID(Y,dY,iE,Yref,dYref,k)

E = Yref - Y;
dE = dYref - dY;

U = k(1)*E + k(2)*iE + k(3)*dE;

== matlab function simulink_motor/motores1/MATLAB Function8 ==
  data: U input; D input; dX output; Y output; X input
function [dX,Y]= motor_modelo(U,D,X)

%MATRICES DEL MOTOR
Ra = 11.24;
La = 2.713e-3;
Kb = 14.87e-3;
Kt = Kb;
bm = 2.01e-6;
Jm = 2779.56e-9;

A = [-Ra/La -Kb/La;Kt/Jm -bm/Jm];
B = [1/La;0];
C = [0 1];

%CONTROLADOR PID
dX = [A*X + B*U];
Y = [C*X + D*U];

== matlab function simulink_motor/motores1/MATLAB Function9 ==
  data: w output; q input; dq input; torque output; ddq input; dw input
function [w,torque] = fcn(q, dq, ddq, dw)

d = [0.2703 0 0.3644 0 0.3743 0 0.2295]; %metros
a = [0.069 0 0.069 0 0.01 0 0]; %matros
alpha = [-pi/2 pi/2 -pi/2 pi/2 -pi/2 pi/2 0]; %radianes
m = [5.70044 3.22698 4.31272 2.07206 2.24665 1.60879 0.54218]; %kg

xc = [-0.05117 0.00269 -0.07176 0.00159 -0.01168 0.00697 0.005137]; %metros
yc = [0.07908 -0.00529 0.08149 -0.01117 0.13111 0.006 0.0009572];
zc = [0.00086 0.06845 0.00132 0.02618 0.0046 0.06048 0.0-6682];

%Tensores de inercia (kg*m^2)
Ixx = [0.047091023 0.027885975 0.026617336 0.013182279 0.016677428 0.007005379 0.000816214];
Iyy = [0.035959884 0.020787492 0.012480083 0.00926852 0.003746311 0.005527552 0.000873501];
Izz = [0.037669765 0.011752094 0.028443552 0.007115827 0.016754573 0.003876072 0.000549415];
Ixy = [-0.0061487 -0.00018822 -0.003921899 -0.000196634 -0.000186576 0.000153481 0.00012844];
Iyx = [-0.0061487 -0.00018822 -0.003921899 -0.000196634 -0.000186576 0.000153481 0.00012844];
Iyz = [-0.000780869 0.002076758 -0.001083893 0.000745949 0.000647324 -0.00021115 0.000105773];
Izy = [-0.000780869 0.002076758 -0.001083893 0.000745949 0.000647324 -0.00021115 0.000105773];
Ixz = [0.000127876 -0.000300964 0.000292706 0.000360362 0.000184037 -0.000443848 0.000189699];
Izx = [0.000127876 -0.000300964 0.000292706 0.000360362 0.000184037 -0.000443848 0.000189699];

Ti = D_H(q,a,alpha,d,0,7);
rici = zeros(3,7);
rmci = zeros(3,7);
rimi = zeros(3,7);

for i = 1:7
    rici(:,i) = Ti{i}(1:3,4)- [xc(i);yc(i);zc(i)];
end

for i = 1:6
    rmci(:,i) = Ti{i + 1}(1:3,4)- Ti{i}(1:3,4) - [xc(i);yc(i);zc(i)];
end

for i = 1:6
    rimi(:,i) = Ti{i + 1}(1:3,4) - Ti{i}(1:3,4);
end

T0 = D_H(q,a,alpha,d,0,7);

w = zeros(3,7);
aw = zeros(3,7);
ac = zeros(3,7);
ae = zeros(3,7);
f = zeros(3,7);
g = zeros(3,7);
Tq = zeros(3,7);
torque = zeros(7,1);

%w1
Ri = Ti{1}(1:3,1:3);
Z0 = [0;0;1];
bi = Ri'*Z0;
w(:,1) = bi*dq(1);
aw(:,1) = bi*ddq(1) + cross(w(:,1),bi*dq(1));
ae(:,1) = cross(dw(:,1),rimi(:,1)) + cross(w(:,1),cross(w(:,1),rimi(:,1)));
ac(:,1) = cross(dw(:,1),rici(:,1)) + cross(w(:,1),cross(w(:,1),rici(:,1)));
g(:,1) = -Ri'*9.78*[0;0;1];

for i = 2:7
   Ri = Ti{i}(1:3,1:3); 
   Rmi = [dot(Ti{i}(1,4),Ti{i-1}(1,4)) dot(Ti{i}(2,4),Ti{i-1}(1,4)) dot(Ti{i}(3,4),Ti{i-1}(1,4));...
       dot(Ti{i}(1,4),Ti{i-1}(2,4)) dot(Ti{i}(2,4),Ti{i-1}(2,4)) dot(Ti{i}(3,4),Ti{i-1}(2,4));...
       dot(Ti{i}(1,4),Ti{i-1}(3,4)) dot(Ti{i}(2,4),Ti{i-1}(3,4)) dot(Ti{i}(3,4),Ti{i-1}(3,4))]';
   bi = Ri'*Ti{i - 1}(1:3,3);
   w(:,i) = Rmi'*w(:,i-1) + bi*dq(i);
   aw(:,i) = Rmi'*aw(:,i-1) +bi*ddq(i) + cross(w(:,i),bi*dq(i));
   ae(:,i) = Rmi'*ae(:,i-1) + cross(dw(:,i),rimi(:,i)) + cross(w(:,i),cross(w(:,i),rimi(:,i)));
   ac(:,i) = Rmi'*ac(:,i-1) + cross(dw(:,i),rici(:,i)) + cross(w(:,i),cross(w(:,i),rici(:,i)));
   g(:,i) = -Ri'*9.78*[0;0;1];
end

%f7
f(:,7) = m(7)*ac(:,7) - m(7)*g(:,7);
I = [Ixx(7) Ixy(7) Ixz(7);Iyx(7) Iyy(7) Iyz(7);Izx(7) Izy(7) Izz(7)];
Tq(:,7) = - cross(f(:,7),rici(:,7)) + aw(:,7) + cross(w(:,7),I*w(:,7));
torque(7) = sqrt(Tq(1,7)^2 + Tq(2,7)^2 + Tq(3,7)^2);

for i = 6:-1:1
    Rmi = [dot(Ti{i + 1}(1,4),Ti{i}(1,4)) dot(Ti{i + 1}(2,4),Ti{i}(1,4)) dot(Ti{i+1}(3,4),Ti{i}(1,4));...
       dot(Ti{i+1}(1,4),Ti{i}(2,4)) dot(Ti{i+1}(2,4),Ti{i}(2,4)) dot(Ti{i+1}(3,4),Ti{i}(2,4));...
       dot(Ti{i+1}(1,4),Ti{i}(3,4)) dot(Ti{i+1}(2,4),Ti{i}(3,4)) dot(Ti{i+1}(3,4),Ti{i}(3,4))]';
   I = [Ixx(i) Ixy(i) Ixz(i);Iyx(i) Iyy(i) Iyz(i);Izx(i) Izy(i) Izz(i)];
   f(:,i) = Rmi*f(:,i+1) + m(i)*ac(:,i) - m(i)*g(:,i);
   Tq(:,i) = Rmi*Tq(:,i+1) - cross(f(:,i),rici(:,i)) + cross(Rmi*f(:,i+1),rmci(:,i)) + aw(:,i) + cross(w(:,i),I*w(:,i));
   torque(i) = sqrt(Tq(1,i)^2 + Tq(2,i)^2 + Tq(3,i)^2);
end
